simulink model "testForEach"  (R2014a)
settings: Solver=FixedStepDiscrete  StartTime=0.0  StopTime=Inf  FixedStep=0.001  RelTol=1e-3
libraries: libButtons x1
settings Model: BufferReuse=off  Creator=djoshea  LastModifiedBy=djoshea
settings SolverCC: EnableConcurrentExecution=on
settings OptimizationCC: BlockReduction=off  OptimizeBlockIOStorage=off  BufferReuse=off  GlobalBufferReuse=off  ExpressionFolding=off  LocalBlockOutputs=off
settings HardwareCC: ProdIntDivRoundTo=Zero  ProdEndianess=LittleEndian  ProdHWDeviceType=Generic->32-bit x86 compatible
settings RTWCC: SystemTargetFile=slrt.tlc  TemplateMakefile=slrt_default_tmf  Description=Simulink Real-Time  ProcessScript=slrt_make_rtw_hook  RTWCompilerOptimization=On
settings SimulinkRealTimeCC: GeneratePreprocessorConditionals=Disable all  EnableShiftOperators=on

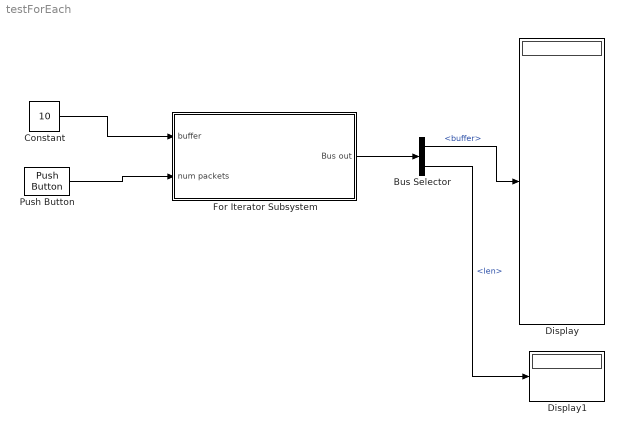
== system testForEach ==
  Bus Selector : BusSelector  OutputSignals=buffer,len
  Constant : Constant  Value=10  OutDataTypeStr=uint8
  Display : Display
  Display1 : Display
  For Iterator Subsystem : Subsystem  TreatAsAtomicUnit=on
  Push Button : libButtons/Push Button  Ts=0.001
  wires:
  Constant/1 -> For Iterator Subsystem/1(buffer)
  Push Button/1 -> For Iterator Subsystem/2(num packets)
  For Iterator Subsystem/1(Bus out) -> Bus Selector/1
  Bus Selector/1 -> Display/1  "<buffer>"
  Bus Selector/2 -> Display1/1  "<len>"

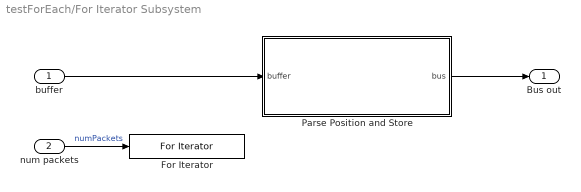
== system testForEach/For Iterator Subsystem ==
  buffer : Inport
  num packets : Inport  Port=2
  For Iterator : ForIterator  IterationSource=external  ShowIterationPort=off  IterationVariableDataType=int8
  Parse Position and Store : MATLAB Function  TreatAsAtomicUnit=on
  Bus out : Outport  OutDataTypeStr=Bus: TestForBus  SourceOfInitialOutputValue=Input signal  InitialOutput=0
  wires:
  num packets/1 -> For Iterator/1  "numPackets"
  Parse Position and Store/1(bus) -> Bus out/1
  buffer/1 -> Parse Position and Store/1(buffer)

== matlab function testForEach/For Iterator Subsystem/Parse Position and Store ==
  data: buffer input uint8 size=1; bus output Bus: TestForBus
function bus = appendToBuffer(buffer)
%#codegen

% generated by BusSerialize.generateCoderVarsizeStatementsForBus('TestForBus', 'pBus');
coder.varsize('pBus.buffer', 100, true);

persistent pBus;
if isempty(pBus)
    pBus = testForEachLib.initializeBus_TestForBus();
end

if numel(pBus.buffer) == 0
    pBus.buffer = buffer;
elseif numel(pBus.buffer) < 100
    pBus.buffer = [pBus.buffer; buffer];
end
pBus.len = uint32(numel(pBus.buffer));

bus = pBus;

end
